simulink model "model_vsi"  (R2020a)
settings: Solver=ode23t  StartTime=0.0  StopTime=t_end  MaxStep=t_step_max  RelTol=solver_tol
values from neighbouring files (symbols this model uses):
  BACK_EMF_DECOUPLING_GAIN = 1    [load_params.m]
  c = 2/3    (= 0.666666666667)    [load_params.m]
  CROSS_COUPLING_DECOUPLING_GAIN = 1    [load_params.m]
  Ke = 0.1    [load_params.m]
  Ki_d = wb_i * R    (= 376.991118431)    [load_params.m]
  Ki_q = wb_i * R    (= 376.991118431)    [load_params.m]
  Kp_d = wb_i * Ld    (= 8.79645943005)    [load_params.m]
  Kp_q = wb_i * Lq    (= 6.28318530718)    [load_params.m]
  Ld = 7e-3    (= 0.007)    [load_params.m]
  Lq = 5e-3    (= 0.005)    [load_params.m]
  OMEGA_E = 2*pi*60    (= 376.991118431)    [load_params.m]
  R = 0.3    [load_params.m]
  V_dc = 200    [load_params.m]
libraries: powerlib_meascontrol x1
settings Model: Creator=Nathan Petersen  LastModifiedBy=Nathan Petersen

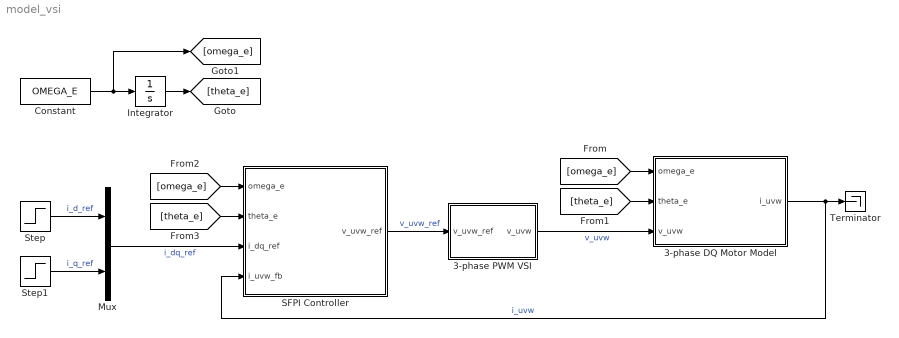
== system model_vsi ==
  3-phase DQ Motor Model : Subsystem
  3-phase PWM VSI : Subsystem
  Constant : Constant  Value=OMEGA_E
  Integrator : Integrator
  Mux : Mux  Inputs=2
  SFPI Controller : Subsystem
  Step : Step  Time=0.1  SampleTime=0
  Step1 : Step  Time=0.2  SampleTime=0
  Terminator : Terminator
  wires:
  Step1/1 -> Mux/2  "i_q_ref"
  Step/1 -> Mux/1  "i_d_ref"
  Constant/1 -> [omega_e], Integrator/1
  Integrator/1 -> [theta_e]
  Mux/1 -> SFPI Controller/3(i_dq_ref)  "i_dq_ref"
  [omega_e] -> 3-phase DQ Motor Model/1(omega_e)
  [theta_e] -> 3-phase DQ Motor Model/2(theta_e)
  3-phase DQ Motor Model/1(i_uvw) -> Terminator/1, SFPI Controller/4(i_uvw_fb)  "i_uvw"
  [omega_e] -> SFPI Controller/1(omega_e)
  [theta_e] -> SFPI Controller/2(theta_e)
  SFPI Controller/1(v_uvw_ref) -> 3-phase PWM VSI/1(v_uvw_ref)  "v_uvw_ref"
  3-phase PWM VSI/1(v_uvw) -> 3-phase DQ Motor Model/3(v_uvw)  "v_uvw"

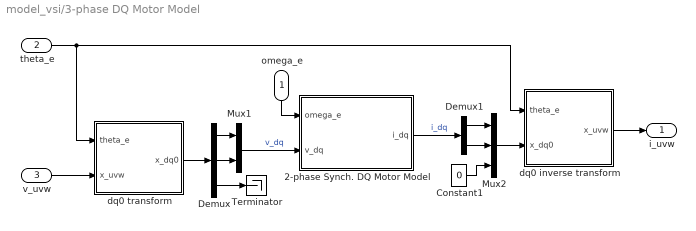
== system model_vsi/3-phase DQ Motor Model ==
  omega_e : Inport
  theta_e : Inport  Port=2
  v_uvw : Inport  Port=3
  2-phase Synch. DQ Motor Model : Subsystem
  Constant1 : Constant  Value=0
  Demux : Demux  Outputs=3
  Demux1 : Demux  Outputs=2
  Mux1 : Mux  Inputs=2
  Mux2 : Mux  Inputs=3
  Terminator : Terminator
  dq0 inverse transform : Subsystem
  dq0 transform : Subsystem
  i_uvw : Outport
  wires:
  Demux1/2 -> Mux2/2
  Demux/1 -> Mux1/1
  Constant1/1 -> Mux2/3
  Mux1/1 -> 2-phase Synch. DQ Motor Model/2(v_dq)  "v_dq"
  Demux1/1 -> Mux2/1
  2-phase Synch. DQ Motor Model/1(i_dq) -> Demux1/1  "i_dq"
  dq0 transform/1(x_dq0) -> Demux/1
  Demux/2 -> Mux1/2
  Mux2/1 -> dq0 inverse transform/2(x_dq0)
  Demux/3 -> Terminator/1
  omega_e/1 -> 2-phase Synch. DQ Motor Model/1(omega_e)
  theta_e/1 -> dq0 transform/1(theta_e), dq0 inverse transform/1(theta_e)
  dq0 inverse transform/1(x_uvw) -> i_uvw/1
  v_uvw/1 -> dq0 transform/2(x_uvw)

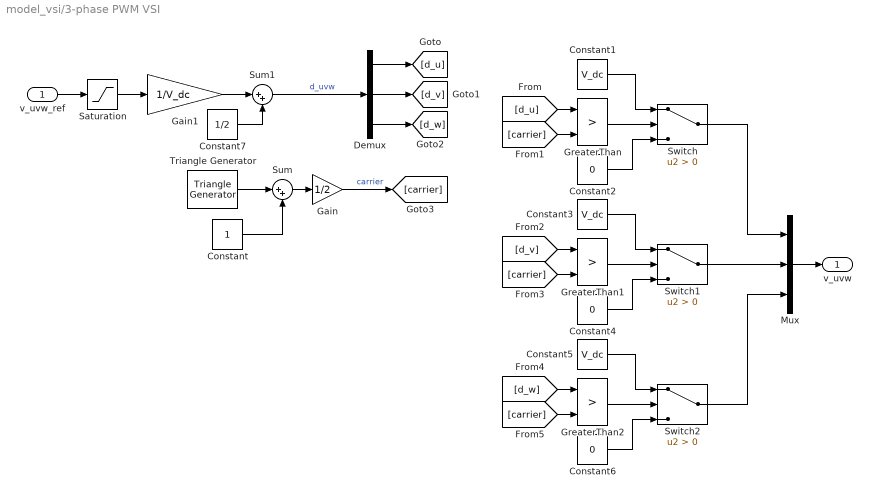
== system model_vsi/3-phase PWM VSI ==
  v_uvw_ref : Inport
  Constant : Constant
  Constant1 : Constant  Value=V_dc
  Constant2 : Constant  Value=0
  Constant3 : Constant  Value=V_dc
  Constant4 : Constant  Value=0
  Constant5 : Constant  Value=V_dc
  Constant6 : Constant  Value=0
  Constant7 : Constant  Value=1/2
  Demux : Demux  Outputs=3
  Gain : Gain  Gain=1/2
  Gain1 : Gain  Gain=1/V_dc
  GreaterThan : RelationalOperator  Operator=>  OutDataTypeStr=boolean  RndMeth=Simplest
  GreaterThan1 : RelationalOperator  Operator=>  OutDataTypeStr=boolean  RndMeth=Simplest
  GreaterThan2 : RelationalOperator  Operator=>  OutDataTypeStr=boolean  RndMeth=Simplest
  Mux : Mux  Inputs=3
  Saturation : Saturate  UpperLimit=+V_dc/2  LowerLimit=-V_dc/2
  Sum : Sum  Inputs=|++
  Sum1 : Sum  Inputs=|++
  Switch : Switch  Criteria=u2 > Threshold
  Switch1 : Switch  Criteria=u2 > Threshold
  Switch2 : Switch  Criteria=u2 > Threshold
  Triangle Generator : powerlib_meascontrol/Pulse & Signal Generators/Triangle Generator  Freq=f_sw  Phase=0  Ts=0
  v_uvw : Outport
  wires:
  Triangle Generator/1 -> Sum/1
  Constant/1 -> Sum/2
  Sum/1 -> Gain/1
  GreaterThan/1 -> Switch/2
  Constant1/1 -> Switch/1
  Constant2/1 -> Switch/3
  Demux/1 -> [d_u]
  Demux/3 -> [d_w]
  Demux/2 -> [d_v]
  Gain/1 -> [carrier]  "carrier"
  [d_u] -> GreaterThan/1
  [carrier] -> GreaterThan/2
  Mux/1 -> v_uvw/1
  Constant4/1 -> Switch1/3
  [carrier] -> GreaterThan1/2
  Constant3/1 -> Switch1/1
  [d_v] -> GreaterThan1/1
  GreaterThan1/1 -> Switch1/2
  Constant6/1 -> Switch2/3
  [carrier] -> GreaterThan2/2
  Constant5/1 -> Switch2/1
  [d_w] -> GreaterThan2/1
  GreaterThan2/1 -> Switch2/2
  Switch/1 -> Mux/1
  Switch1/1 -> Mux/2
  Switch2/1 -> Mux/3
  Gain1/1 -> Sum1/1
  Sum1/1 -> Demux/1  "d_uvw"
  Constant7/1 -> Sum1/2
  Saturation/1 -> Gain1/1
  v_uvw_ref/1 -> Saturation/1

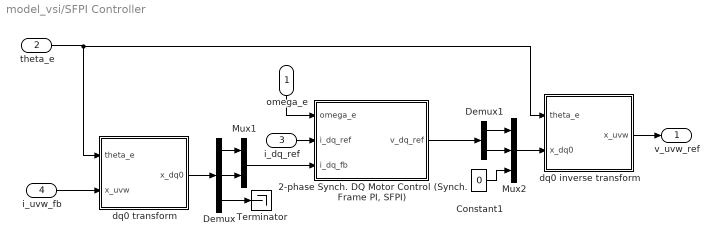
== system model_vsi/SFPI Controller ==
  omega_e : Inport
  theta_e : Inport  Port=2
  i_dq_ref : Inport  Port=3
  i_uvw_fb : Inport  Port=4
  "2-phase Synch. DQ Motor Control (Synch. Frame PI, SFPI)" : Subsystem
  Constant1 : Constant  Value=0
  Demux : Demux  Outputs=3
  Demux1 : Demux  Outputs=2
  Mux1 : Mux  Inputs=2
  Mux2 : Mux  Inputs=3
  Terminator : Terminator
  dq0 inverse transform : Subsystem
  dq0 transform : Subsystem
  v_uvw_ref : Outport
  wires:
  Demux/3 -> Terminator/1
  Demux/1 -> Mux1/1
  Demux/2 -> Mux1/2
  Demux1/1 -> Mux2/1
  Mux2/1 -> dq0 inverse transform/2(x_dq0)
  Demux1/2 -> Mux2/2
  Constant1/1 -> Mux2/3
  theta_e/1 -> dq0 transform/1(theta_e), dq0 inverse transform/1(theta_e)
  dq0 transform/1(x_dq0) -> Demux/1
  "2-phase Synch. DQ Motor Control (Synch. Frame PI, SFPI)"/1(v_dq_ref) -> Demux1/1
  Mux1/1 -> "2-phase Synch. DQ Motor Control (Synch. Frame PI, SFPI)"/3(i_dq_fb)
  omega_e/1 -> "2-phase Synch. DQ Motor Control (Synch. Frame PI, SFPI)"/1(omega_e)
  dq0 inverse transform/1(x_uvw) -> v_uvw_ref/1
  i_uvw_fb/1 -> dq0 transform/2(x_uvw)
  i_dq_ref/1 -> "2-phase Synch. DQ Motor Control (Synch. Frame PI, SFPI)"/2(i_dq_ref)

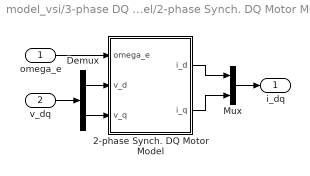
== system model_vsi/3-phase DQ Motor Model/2-phase Synch. DQ Motor Model ==
  omega_e : Inport
  v_dq : Inport  Port=2
  2-phase Synch. DQ Motor Model : Subsystem
  Demux : Demux  Outputs=2
  Mux : Mux  Inputs=2
  i_dq : Outport
  wires:
  v_dq/1 -> Demux/1
  Demux/2 -> 2-phase Synch. DQ Motor Model/3(v_q)
  Demux/1 -> 2-phase Synch. DQ Motor Model/2(v_d)
  omega_e/1 -> 2-phase Synch. DQ Motor Model/1(omega_e)
  2-phase Synch. DQ Motor Model/1(i_d) -> Mux/1
  2-phase Synch. DQ Motor Model/2(i_q) -> Mux/2
  Mux/1 -> i_dq/1

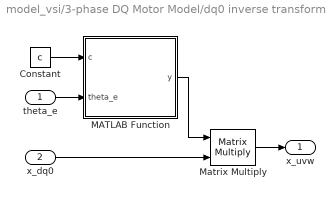
== system model_vsi/3-phase DQ Motor Model/dq0 inverse transform ==
  theta_e : Inport
  x_dq0 : Inport  Port=2
  Constant : Constant  Value=c
  MATLAB Function : MATLAB Function  TreatAsAtomicUnit=on
  Matrix Multiply : Product  Multiplication=Matrix(*)
  x_uvw : Outport
  wires:
  Matrix Multiply/1 -> x_uvw/1
  MATLAB Function/1(y) -> Matrix Multiply/1
  x_dq0/1 -> Matrix Multiply/2
  theta_e/1 -> MATLAB Function/2(theta_e)
  Constant/1 -> MATLAB Function/1(c)

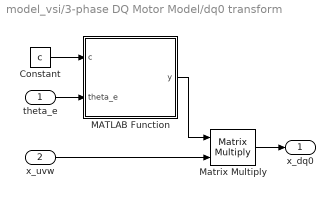
== system model_vsi/3-phase DQ Motor Model/dq0 transform ==
  theta_e : Inport
  x_uvw : Inport  Port=2
  Constant : Constant  Value=c
  MATLAB Function : MATLAB Function  TreatAsAtomicUnit=on
  Matrix Multiply : Product  Multiplication=Matrix(*)
  x_dq0 : Outport
  wires:
  x_uvw/1 -> Matrix Multiply/2
  theta_e/1 -> MATLAB Function/2(theta_e)
  Constant/1 -> MATLAB Function/1(c)
  MATLAB Function/1(y) -> Matrix Multiply/1
  Matrix Multiply/1 -> x_dq0/1

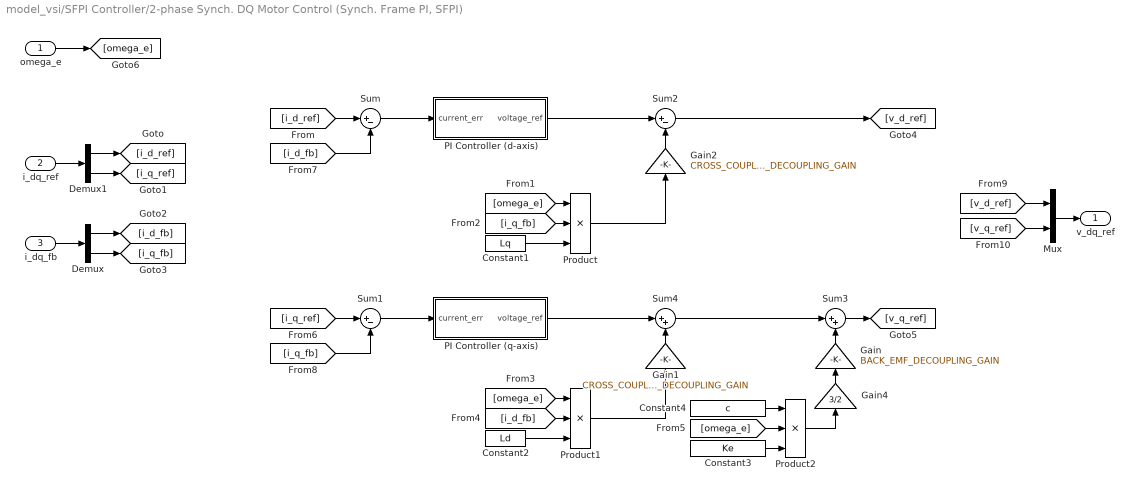
== system model_vsi/SFPI Controller/2-phase Synch. DQ Motor Control (Synch. Frame PI, SFPI) ==
  omega_e : Inport
  i_dq_ref : Inport  Port=2
  i_dq_fb : Inport  Port=3
  Constant1 : Constant  Value=Lq
  Constant2 : Constant  Value=Ld
  Constant3 : Constant  Value=Ke
  Constant4 : Constant  Value=c
  Demux : Demux  Outputs=2
  Demux1 : Demux  Outputs=2
  Gain : Gain  Gain=BACK_EMF_DECOUPLING_GAIN
  Gain1 : Gain  Gain=CROSS_COUPLING_DECOUPLING_GAIN
  Gain2 : Gain  Gain=CROSS_COUPLING_DECOUPLING_GAIN
  Gain4 : Gain  Gain=3/2
  Mux : Mux  Inputs=2
  PI Controller (d-axis) : Subsystem
  PI Controller (q-axis) : Subsystem
  Product : Product  Inputs=3
  Product1 : Product  Inputs=3
  Product2 : Product  Inputs=3
  Sum : Sum  Inputs=|+-
  Sum1 : Sum  Inputs=|+-
  Sum2 : Sum  Inputs=|+-
  Sum3 : Sum  Inputs=|++
  Sum4 : Sum  Inputs=|++
  v_dq_ref : Outport
  wires:
  Constant3/1 -> Product2/3
  Product/1 -> Gain2/1
  Sum/1 -> PI Controller (d-axis)/1(current_err)
  [omega_e] -> Product/1
  Sum2/1 -> [v_d_ref]
  PI Controller (d-axis)/1(voltage_ref) -> Sum2/1
  PI Controller (q-axis)/1(voltage_ref) -> Sum4/1
  [i_q_fb] -> Product/2
  Constant1/1 -> Product/3
  Constant4/1 -> Product2/1
  Product2/1 -> Gain4/1
  [i_d_fb] -> Product1/2
  Sum4/1 -> Sum3/1
  Constant2/1 -> Product1/3
  Product1/1 -> Gain1/1
  [omega_e] -> Product2/2
  Gain/1 -> Sum3/2
  Gain2/1 -> Sum2/2
  Gain1/1 -> Sum4/2
  Gain4/1 -> Gain/1
  Sum1/1 -> PI Controller (q-axis)/1(current_err)
  [omega_e] -> Product1/1
  Sum3/1 -> [v_q_ref]
  i_dq_fb/1 -> Demux/1
  i_dq_ref/1 -> Demux1/1
  Demux1/1 -> [i_d_ref]
  Demux1/2 -> [i_q_ref]
  Demux/2 -> [i_q_fb]
  Demux/1 -> [i_d_fb]
  [i_q_ref] -> Sum1/1
  [i_d_ref] -> Sum/1
  [i_d_fb] -> Sum/2
  [i_q_fb] -> Sum1/2
  [v_d_ref] -> Mux/1
  [v_q_ref] -> Mux/2
  Mux/1 -> v_dq_ref/1
  omega_e/1 -> [omega_e]

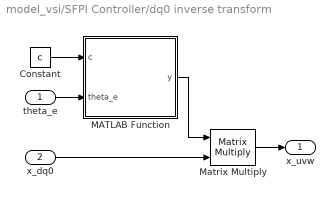
== system model_vsi/SFPI Controller/dq0 inverse transform ==
  theta_e : Inport
  x_dq0 : Inport  Port=2
  Constant : Constant  Value=c
  MATLAB Function : MATLAB Function  TreatAsAtomicUnit=on
  Matrix Multiply : Product  Multiplication=Matrix(*)
  x_uvw : Outport
  wires:
  Matrix Multiply/1 -> x_uvw/1
  MATLAB Function/1(y) -> Matrix Multiply/1
  x_dq0/1 -> Matrix Multiply/2
  theta_e/1 -> MATLAB Function/2(theta_e)
  Constant/1 -> MATLAB Function/1(c)

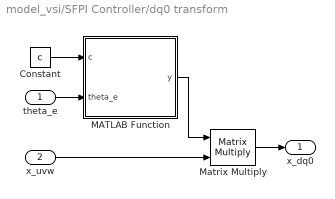
== system model_vsi/SFPI Controller/dq0 transform ==
  theta_e : Inport
  x_uvw : Inport  Port=2
  Constant : Constant  Value=c
  MATLAB Function : MATLAB Function  TreatAsAtomicUnit=on
  Matrix Multiply : Product  Multiplication=Matrix(*)
  x_dq0 : Outport
  wires:
  x_uvw/1 -> Matrix Multiply/2
  theta_e/1 -> MATLAB Function/2(theta_e)
  Constant/1 -> MATLAB Function/1(c)
  MATLAB Function/1(y) -> Matrix Multiply/1
  Matrix Multiply/1 -> x_dq0/1

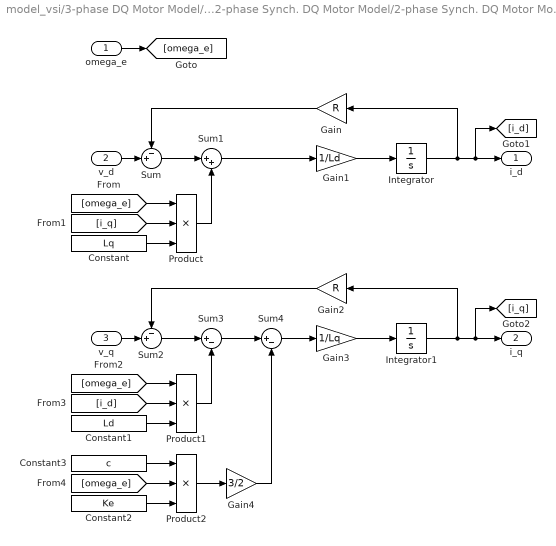
== system model_vsi/3-phase DQ Motor Model/2-phase Synch. DQ Motor Model/2-phase Synch. DQ Motor Model ==
  omega_e : Inport
  v_d : Inport  Port=2
  v_q : Inport  Port=3
  Constant : Constant  Value=Lq
  Constant1 : Constant  Value=Ld
  Constant2 : Constant  Value=Ke
  Constant3 : Constant  Value=c
  Gain : Gain  Gain=R
  Gain1 : Gain  Gain=1/Ld
  Gain2 : Gain  Gain=R
  Gain3 : Gain  Gain=1/Lq
  Gain4 : Gain  Gain=3/2
  Integrator : Integrator
  Integrator1 : Integrator
  Product : Product  Inputs=3
  Product1 : Product  Inputs=3
  Product2 : Product  Inputs=3
  Sum : Sum  Inputs=-+|
  Sum1 : Sum  Inputs=|++
  Sum2 : Sum  Inputs=-+|
  Sum3 : Sum  Inputs=|+-
  Sum4 : Sum  Inputs=|+-
  i_d : Outport
  i_q : Outport  Port=2
  wires:
  Gain1/1 -> Integrator/1
  Integrator/1 -> [i_d], i_d/1, Gain/1
  v_d/1 -> Sum/2
  Gain/1 -> Sum/1
  Sum/1 -> Sum1/1
  Product/1 -> Sum1/2
  [omega_e] -> Product/1
  [i_q] -> Product/2
  Constant/1 -> Product/3
  omega_e/1 -> [omega_e]
  Sum1/1 -> Gain1/1
  Constant1/1 -> Product1/3
  Gain2/1 -> Sum2/1
  v_q/1 -> Sum2/2
  Product1/1 -> Sum3/2
  [omega_e] -> Product1/1
  Sum2/1 -> Sum3/1
  Integrator1/1 -> [i_q], i_q/1, Gain2/1
  Gain3/1 -> Integrator1/1
  [i_d] -> Product1/2
  Sum3/1 -> Sum4/1
  Sum4/1 -> Gain3/1
  [omega_e] -> Product2/2
  Constant2/1 -> Product2/3
  Product2/1 -> Gain4/1
  Constant3/1 -> Product2/1
  Gain4/1 -> Sum4/2

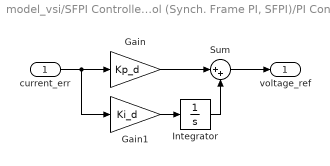
== system model_vsi/SFPI Controller/2-phase Synch. DQ Motor Control (Synch. Frame PI, SFPI)/PI Controller (d-axis) ==
  current_err : Inport
  Gain : Gain  Gain=Kp_d
  Gain1 : Gain  Gain=Ki_d
  Integrator : Integrator
  Sum : Sum  Inputs=|++
  voltage_ref : Outport
  wires:
  current_err/1 -> Gain1/1, Gain/1
  Gain/1 -> Sum/1
  Sum/1 -> voltage_ref/1
  Gain1/1 -> Integrator/1
  Integrator/1 -> Sum/2

== system model_vsi/SFPI Controller/2-phase Synch. DQ Motor Control (Synch. Frame PI, SFPI)/PI Controller (q-axis) ==
  current_err : Inport
  Gain : Gain  Gain=Kp_q
  Gain1 : Gain  Gain=Ki_q
  Integrator : Integrator
  Sum : Sum  Inputs=|++
  voltage_ref : Outport
  wires:
  current_err/1 -> Gain1/1, Gain/1
  Gain/1 -> Sum/1
  Sum/1 -> voltage_ref/1
  Gain1/1 -> Integrator/1
  Integrator/1 -> Sum/2

== matlab function model_vsi/3-phase DQ Motor Model/dq0 transform/MATLAB Function ==
  data: c input; theta_e input; y output
function y = C_R(c, theta_e)

y = c .* [
     cos(theta_e),  cos(theta_e - 2*pi/3),  cos(theta_e - 4*pi/3);
    -sin(theta_e), -sin(theta_e - 2*pi/3), -sin(theta_e - 4*pi/3);
          1/(3*c),                1/(3*c),                1/(3*c);
];

end

== matlab function model_vsi/SFPI Controller/dq0 inverse transform/MATLAB Function ==
  data: c input; theta_e input; y output
function y = C_R_inv(c, theta_e)

y = (2/(3*c)) .* [
    cos(theta_e),             -sin(theta_e),           3*c/2;
    cos(theta_e + 4*pi/3),    -sin(theta_e + 4*pi/3),  3*c/2;
    cos(theta_e + 2*pi/3),    -sin(theta_e + 2*pi/3),  3*c/2;
];

end

== matlab function model_vsi/SFPI Controller/dq0 transform/MATLAB Function ==
  data: c input; theta_e input; y output
function y = C_R(c, theta_e)

y = c .* [
     cos(theta_e),  cos(theta_e - 2*pi/3),  cos(theta_e - 4*pi/3);
    -sin(theta_e), -sin(theta_e - 2*pi/3), -sin(theta_e - 4*pi/3);
          1/(3*c),                1/(3*c),                1/(3*c);
];

end

== matlab function model_vsi/3-phase DQ Motor Model/dq0 inverse transform/MATLAB Function ==
  data: c input; theta_e input; y output
function y = C_R_inv(c, theta_e)

y = (2/(3*c)) .* [
    cos(theta_e),             -sin(theta_e),           3*c/2;
    cos(theta_e + 4*pi/3),    -sin(theta_e + 4*pi/3),  3*c/2;
    cos(theta_e + 2*pi/3),    -sin(theta_e + 2*pi/3),  3*c/2;
];

end
